simulink model "sltestThrottlePositionMonitorMdlRef"  (R2023a)
settings: Solver=FixedStepDiscrete  StartTime=0.0  StopTime=10.0  FixedStep=0.005  RelTol=1e-3
PreLoadFcn:
  | Simulink.defineIntEnumType('SensorOption',...
  |     {'Primary', 'Secondary'},...
  |     [0;1],...
  |     'DefaultValue', 'Primary');
  | 
  | SensorSelection = Simulink.Parameter;
  | SensorSelection.Value = SensorOption.Primary;
  | SensorSelection.DataType = 'Enum: SensorOption';
undefined symbols (not defined in the file): SensorOption
libraries: simulink x1
settings Model: Creator=The MathWorks, Inc.  LastModifiedBy=The MathWorks, Inc.
settings SolverCC: AlgebraicLoopSolver=TrustRegion  MaxZcPerStep=1
settings DataIOCC: SaveFormat=StructureWithTime  ReturnWorkspaceOutputs=off
settings OptimizationCC: DefaultParameterBehavior=Inlined  PassReuseOutputArgsAs=Individual arguments  ZeroExternalMemoryAtStartup=off  ZeroInternalMemoryAtStartup=off  EfficientTunableParamExpr=on
settings DebuggingCC: ParameterTunabilityLossMsg=error  UnconnectedInputMsg=warning  UnconnectedOutputMsg=warning  UnconnectedLineMsg=warning  ArithmeticOperatorsInVariantConditions=warning
settings ModelReferenceCC: EnableRefExpFcnMdlSchedulingChecks=on
settings SFSimCC: SimUseLocalCustomCode=off  MATLABDynamicMemAlloc=off  CustomCodeUndefinedFunction=UseInterfaceOnly
settings RTWCC: Description=AUTOSAR  SystemTargetFile=autosar.tlc  GenCodeOnly=on  TemplateMakefile=ert_default_tmf  GenerateReport=on  RTWUseLocalCustomCode=off  IncludeHyperlinkInReport=on  LaunchReport=on  PortableWordSizes=on  GenerateTraceInfo=on  GenerateTraceReport=on  GenerateTraceReportSl=on  GenerateTraceReportSf=on  GenerateTraceReportEml=on  DLArmComputeVersion=19.05
settings CodeAppCC: ForceParamTrailComments=on  IgnoreCustomStorageClasses=off  OperatorAnnotations=on  SimulinkDataObjDesc=on  SFDataObjDesc=on  InsertBlockDesc=on
settings STFCustomTargetCC: MultiwordLength=256  ParMdlRefBuildCompliant=on  CompOptLevelCompliant=on  ConcurrentExecutionCompliant=off  IncludeMdlTerminateFcn=off  CombineOutputUpdateFcns=on  SuppressErrorStatus=on  ERTCustomFileBanners=on  SupportNonFinite=off  SupportComplex=off  SupportContinuousTime=off  SupportNonInlinedSFcns=off  RemoveResetFunc=on  MATLABClassNameForMDSCustomization=Simulink.SoftwareTarget.ERTCustomization  AutosarCompliant=on  GRTInterface=off  LookupTableObjectStructAxisOrder=2,1,3,4,...  LUTObjectStructOrderEvenSpacing=Size,Table,Breakpoints  SystemTargetFile=autosar.tlc
settings ERTTargetCC: TargetLangStandard=C99 (ISO)  ConcurrentExecutionCompliant=off  IncludeMdlTerminateFcn=off  SuppressErrorStatus=on  SupportNonFinite=off  SupportComplex=off  ModelStepFunctionPrototypeControlCompliant=off  CPPClassGenCompliant=off  AutosarCompliant=on  LookupTableObjectStructAxisOrder=2,1,3,4,...  LUTObjectStructOrderEvenSpacing=Size,Table,Breakpoints  InlinedParameterPlacement=NonHierarchical  ERTCustomFileTemplate=example_file_process.tlc

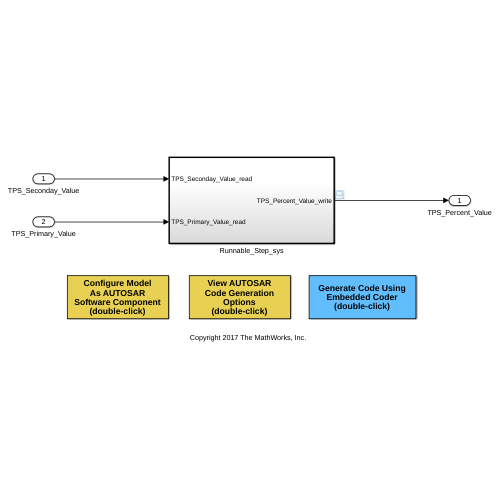
[thumbnail: Simulink's stored preview of the top-level diagram]
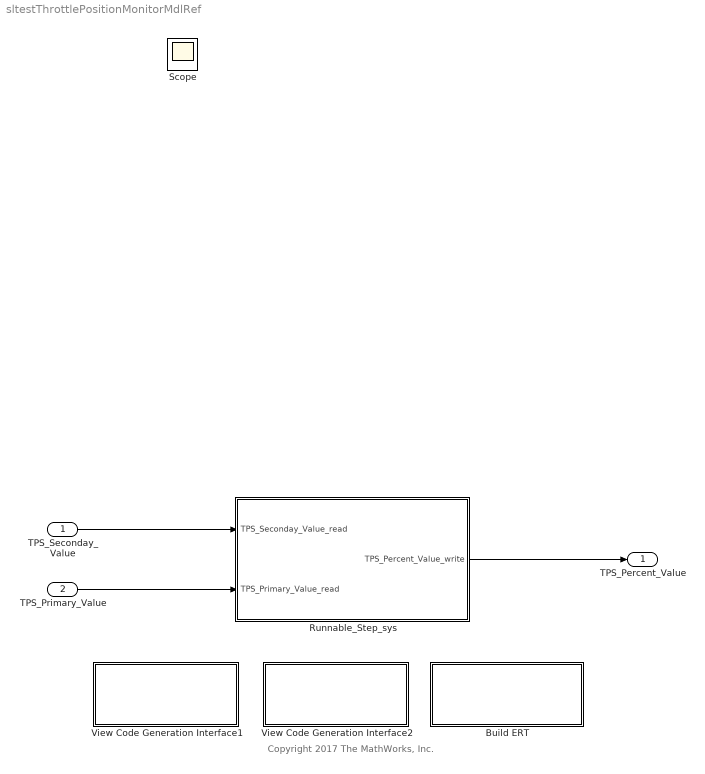
== system sltestThrottlePositionMonitorMdlRef ==
  note: Copyright 2017 The MathWorks, Inc.
  TPS_Seconday_Value : Inport  OutDataTypeStr=single  PortDimensions=1
  TPS_Primary_Value : Inport  Port=2  OutDataTypeStr=single  PortDimensions=1
  Build ERT : Subsystem  mask{attrib_overrides={'RTWCAPIParams','RTWCAPISignals','RTWCAPIStates'}}
      mask prompts: attrib_overrides "List of attributes to preserve (cell of strings):"
      mask help: Enter the attributes of the configuration set that you want preserved. Otherwise, the default configuration script will override your current settings.
      settings: OpenFcn=|
      | try
      |     if ~exist('rtwdemo_ert', 'dir')
      |         disp('Creating working directory rtwdemo_ert')
      |         mkdir('rtwdemo_ert')
      |     end
      |     cd('rtwdemo_ert');
      |     rtwbuilddemomodel(bdroot);
      |     cd('..');
      | catch myException
      |     rethrow(myException);
      | end
      mask Display:
      | disp(['Generate Code Using\n',...
      | 	 'Embedded Coder\n'...
      | 	  '(double-click)'])
  Runnable_Step_sys : Subsystem  TreatAsAtomicUnit=on  SystemSampleTime=0.005
  View Code Generation Interface1 : Subsystem
      settings: OpenFcn=autosar_ui_launch(bdroot)
      mask Display: disp('Configure Model\nAs AUTOSAR\nSoftware Component\n(double-click)')
  View Code Generation Interface2 : Subsystem
      settings: OpenFcn=|
      | dlg = slCfgPrmDlg(bdroot,'Open');
      | dlg = slCfgPrmDlg(bdroot,'TurnToPage',[message('RTW:configSet:configSetCodeGen').getString,'/',message('RTW:autosar:autosarCodeGenOptions').getString]);
      | clear dlg;
      mask Display: disp('View AUTOSAR\nCode Generation\nOptions\n(double-click)')
  TPS_Percent_Value : Outport  OutDataTypeStr=single  PortDimensions=1  VectorParamsAs1DForOutWhenUnconnected=off
  Scope : Scope
  wires:
  TPS_Seconday_Value/1 -> Runnable_Step_sys/1(TPS_Seconday_Value_read)
  TPS_Primary_Value/1 -> Runnable_Step_sys/2(TPS_Primary_Value_read)
  Runnable_Step_sys/1(TPS_Percent_Value_write) -> TPS_Percent_Value/1

== system sltestThrottlePositionMonitorMdlRef/Build ERT ==

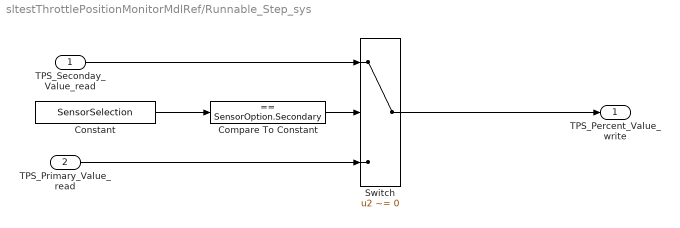
== system sltestThrottlePositionMonitorMdlRef/Runnable_Step_sys ==
  TPS_Seconday_Value_read : Inport
  TPS_Primary_Value_read : Inport  Port=2
  Compare To Constant : simulink/Logic and Bit Operations/Compare To Constant  relop===  const=SensorOption.Secondary  OutDataTypeStr=boolean
  Constant : Constant  Value=SensorSelection
  Switch : Switch  Criteria=u2 ~= 0  SaturateOnIntegerOverflow=off  InputSameDT=off
  TPS_Percent_Value_write : Outport  VectorParamsAs1DForOutWhenUnconnected=off
  wires:
  TPS_Seconday_Value_read/1 -> Switch/1
  TPS_Primary_Value_read/1 -> Switch/3
  Switch/1 -> TPS_Percent_Value_write/1
  Constant/1 -> Compare To Constant/1
  Compare To Constant/1 -> Switch/2

== system sltestThrottlePositionMonitorMdlRef/View Code Generation Interface1 ==

== system sltestThrottlePositionMonitorMdlRef/View Code Generation Interface2 ==
